simulink model "Model (1)"  (R2020a)
settings: Solver=VariableStepAuto  StartTime=0.0  StopTime=10.0  RelTol=1e-3
libraries: dspsigops x3, dsparch4 x3, dspswit3 x1, simulink_extras x1
settings Model: Creator=User  LastModifiedBy=Madhura

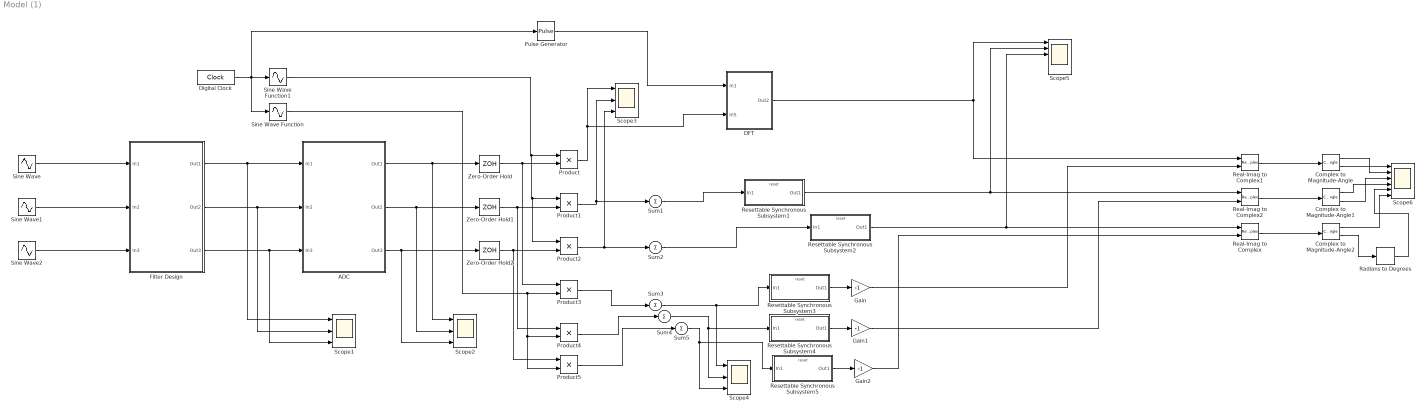
== system Model (1) ==
  ADC : Subsystem
  Complex to Magnitude-Angle : ComplexToMagnitudeAngle
  Complex to Magnitude-Angle1 : ComplexToMagnitudeAngle
  Complex to Magnitude-Angle2 : ComplexToMagnitudeAngle
  DFT : Subsystem
  Digital Clock : DigitalClock  SampleTime=0.001
  Filter Design : Subsystem
  Gain : Gain  Gain=-1
  Gain1 : Gain  Gain=-1
  Gain2 : Gain  Gain=-1
  Product{,1..5} (6 alike) : Product
  Pulse Generator : DiscretePulseGenerator  PulseType=Time based  TimeSource=Use external signal  Period=0.04  PulseWidth=50
  Radians to Degrees : simulink_extras/Transformations/Radians to Degrees
  Real-Imag to Complex : RealImagToComplex
  Real-Imag to Complex1 : RealImagToComplex
  Real-Imag to Complex2 : RealImagToComplex
  Resettable Synchronous Subsystem1 : Subsystem  TreatAsAtomicUnit=on
  Resettable Synchronous Subsystem2 : Subsystem  TreatAsAtomicUnit=on
  Resettable Synchronous Subsystem3 : Subsystem  TreatAsAtomicUnit=on
  Resettable Synchronous Subsystem4 : Subsystem  TreatAsAtomicUnit=on
  Resettable Synchronous Subsystem5 : Subsystem  TreatAsAtomicUnit=on
  Scope{1..4} (4 alike) : Scope  NumInputPorts=3
  Scope5 : Scope  NumInputPorts=6
  Scope6 : Scope  NumInputPorts=6
  Sine Wave : Sin  Amplitude=1.5  Frequency=2*pi*(53)  SampleTime=0
  Sine Wave Function : Sin  TimeSource=Use external signal  Frequency=2*pi/20  SampleTime=0
  Sine Wave Function1 : Sin  TimeSource=Use external signal  Frequency=2*pi/20  Phase=pi/2  SampleTime=0
  Sine Wave1 : Sin  Frequency=2*pi*50  SampleTime=0
  Sine Wave2 : Sin  Frequency=2*pi*50  Phase=-2*pi/3  SampleTime=0
  Sum1 : Sum  Inputs=+  CollapseMode=Specified dimension
  Sum{2..5} (4 alike) : Sum  Inputs=+
  Zero-Order Hold : ZeroOrderHold  SampleTime=-1
  Zero-Order Hold1 : ZeroOrderHold  SampleTime=-1
  Zero-Order Hold2 : ZeroOrderHold  SampleTime=-1
  wires:
  Sine Wave/1 -> Filter Design/1(In1)
  ADC/2(Out2) -> Zero-Order Hold1/1, Scope2/2
  Sine Wave1/1 -> Filter Design/2(In2)
  Filter Design/1(Out1) -> Scope1/1, ADC/1(In1)
  ADC/3(Out3) -> Zero-Order Hold2/1, Scope2/3
  ADC/1(Out1) -> Zero-Order Hold/1, Scope2/1
  Sine Wave2/1 -> Filter Design/3(In3)
  Filter Design/2(Out2) -> Scope1/2, ADC/2(In2)
  Filter Design/3(Out3) -> Scope1/3, ADC/3(In3)
  Zero-Order Hold/1 -> Product3/1, Product/2
  Zero-Order Hold1/1 -> Product4/1, Product1/2
  Zero-Order Hold2/1 -> Product5/1, Product2/2
  Digital Clock/1 -> Pulse Generator/1, Sine Wave Function1/1, Sine Wave Function/1
  Sine Wave Function1/1 -> Product2/1, Product1/1, Product/1
  Product1/1 -> Sum1/1, Scope3/2
  Product2/1 -> Sum2/1, Scope3/3
  Sine Wave Function/1 -> Product5/2, Product4/2, Product3/2
  Product3/1 -> Sum3/1
  Product4/1 -> Sum4/1
  Product5/1 -> Sum5/1
  Product/1 -> DFT/2(In5), Scope3/1
  Sum3/1 -> Resettable Synchronous Subsystem3/1(In1), Scope4/1
  Sum4/1 -> Resettable Synchronous Subsystem4/1(In1), Scope4/2
  Sum5/1 -> Resettable Synchronous Subsystem5/1(In1), Scope4/3
  Gain/1 -> Real-Imag to Complex1/2
  Gain1/1 -> Real-Imag to Complex2/2
  Gain2/1 -> Real-Imag to Complex/2
  Real-Imag to Complex1/1 -> Complex to Magnitude-Angle/1
  Real-Imag to Complex2/1 -> Complex to Magnitude-Angle1/1
  Real-Imag to Complex/1 -> Complex to Magnitude-Angle2/1
  Complex to Magnitude-Angle/2 -> Scope6/1
  Complex to Magnitude-Angle1/2 -> Scope6/3
  Complex to Magnitude-Angle/1 -> Scope6/2
  Complex to Magnitude-Angle1/1 -> Scope6/4
  Complex to Magnitude-Angle2/1 -> Scope6/6
  Resettable Synchronous Subsystem3/1(Out1) -> Gain/1
  Resettable Synchronous Subsystem1/1(Out1) -> Scope5/2, Real-Imag to Complex2/1
  Sum1/1 -> Resettable Synchronous Subsystem1/1(In1)
  Sum2/1 -> Resettable Synchronous Subsystem2/1(In1)
  Resettable Synchronous Subsystem2/1(Out1) -> Scope5/3, Real-Imag to Complex/1
  Resettable Synchronous Subsystem4/1(Out1) -> Gain1/1
  Resettable Synchronous Subsystem5/1(Out1) -> Gain2/1
  Complex to Magnitude-Angle2/2 -> Radians to Degrees/1
  Radians to Degrees/1 -> Scope6/5
  DFT/1(Out2) -> Scope5/1, Real-Imag to Complex1/1
  Pulse Generator/1 -> DFT/1(In1)

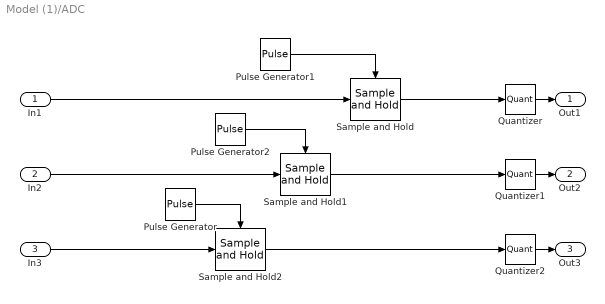
== system Model (1)/ADC ==
  In1 : Inport
  In2 : Inport  Port=2
  In3 : Inport  Port=3
  Pulse Generator : DiscretePulseGenerator  PulseType=Time based  Period=0.001  PulseWidth=5
  Pulse Generator1 : DiscretePulseGenerator  PulseType=Time based  Period=0.001  PulseWidth=5
  Pulse Generator2 : DiscretePulseGenerator  PulseType=Time based  Period=0.001  PulseWidth=5
  Quantizer : Quantizer  QuantizationInterval=0.1
  Quantizer1 : Quantizer  QuantizationInterval=0.1
  Quantizer2 : Quantizer  QuantizationInterval=0.1
  Sample and Hold : dspsigops/Sample and Hold  trig=Rising edge  initCond=0  latchinput=off
  Sample and Hold1 : dspsigops/Sample and Hold  trig=Rising edge  initCond=0  latchinput=off
  Sample and Hold2 : dspsigops/Sample and Hold  trig=Rising edge  initCond=0  latchinput=off
  Out1 : Outport
  Out2 : Outport  Port=2
  Out3 : Outport  Port=3
  wires:
  In1/1 -> Sample and Hold/1
  Sample and Hold2/1 -> Quantizer2/1
  Sample and Hold1/1 -> Quantizer1/1
  Pulse Generator1/1 -> Sample and Hold/Trigger
  In2/1 -> Sample and Hold1/1
  Pulse Generator/1 -> Sample and Hold2/Trigger
  Quantizer2/1 -> Out3/1
  Sample and Hold/1 -> Quantizer/1
  Pulse Generator2/1 -> Sample and Hold1/Trigger
  Quantizer/1 -> Out1/1
  Quantizer1/1 -> Out2/1
  In3/1 -> Sample and Hold2/1

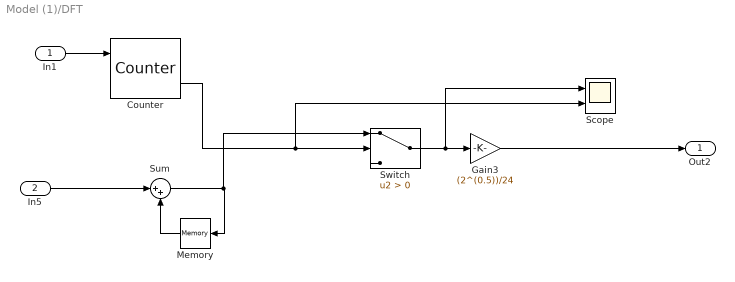
== system Model (1)/DFT ==
  In1 : Inport
  In5 : Inport  Port=2
  Counter : dspswit3/Counter  Direction=Up  CountEvent=Rising edge  CounterSize=User defined  MaxCount=20  InitialCount=0  Output=Count and Hit  HitValue=20  ResetInput=on  SamplesPerFrame=1  Ts=1  CntDtype=double  HitDtype=Logical
  Gain3 : Gain  Gain=(2^(0.5))/24
  Memory : Memory
  Scope : Scope  NumInputPorts=2
  Sum : Sum  Inputs=|++
  Switch : Switch  Criteria=u2 > Threshold
  Out2 : Outport
  wires:
  Gain3/1 -> Out2/1
  Switch/1 -> Scope/1, Gain3/1
  Sum/1 -> Switch/1, Memory/1
  In1/1 -> Counter/1
  Memory/1 -> Sum/2
  In5/1 -> Sum/1
  Counter/2 -> Scope/2, Switch/2

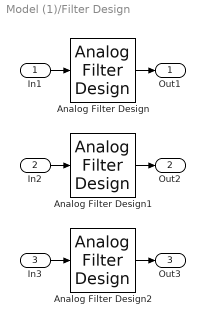
== system Model (1)/Filter Design ==
  In1 : Inport
  In2 : Inport  Port=2
  In3 : Inport  Port=3
  Analog Filter Design : dsparch4/Analog Filter Design  method=Butterworth  filttype=Lowpass  N=8  Wlo=2*pi*60  Whi=80  Rp=2  Rs=40
  Analog Filter Design1 : dsparch4/Analog Filter Design  method=Butterworth  filttype=Lowpass  N=8  Wlo=2*pi*60  Whi=80  Rp=2  Rs=40
  Analog Filter Design2 : dsparch4/Analog Filter Design  method=Butterworth  filttype=Lowpass  N=8  Wlo=2*pi*60  Whi=80  Rp=2  Rs=40
  Out1 : Outport
  Out2 : Outport  Port=2
  Out3 : Outport  Port=3
  wires:
  In2/1 -> Analog Filter Design1/1
  Analog Filter Design1/1 -> Out2/1
  In1/1 -> Analog Filter Design/1
  Analog Filter Design2/1 -> Out3/1
  In3/1 -> Analog Filter Design2/1
  Analog Filter Design/1 -> Out1/1

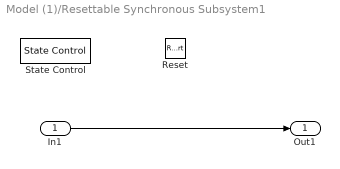
== system Model (1)/Resettable Synchronous Subsystem1 ==
  In1 : Inport
  Reset : ResetPort  DisableCoverage=on  ResetTriggerType=level hold
  State Control : StateControl  StateControl=Synchronous
  Out1 : Outport  VectorParamsAs1DForOutWhenUnconnected=off
  wires:
  In1/1 -> Out1/1

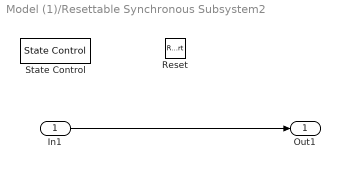
== system Model (1)/Resettable Synchronous Subsystem2 ==
  In1 : Inport
  Reset : ResetPort  DisableCoverage=on  ResetTriggerType=level hold
  State Control : StateControl  StateControl=Synchronous
  Out1 : Outport  VectorParamsAs1DForOutWhenUnconnected=off
  wires:
  In1/1 -> Out1/1

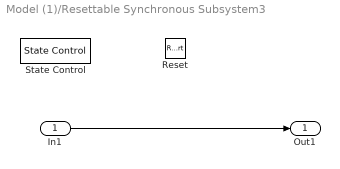
== system Model (1)/Resettable Synchronous Subsystem3 ==
  In1 : Inport
  Reset : ResetPort  DisableCoverage=on  ResetTriggerType=level hold
  State Control : StateControl  StateControl=Synchronous
  Out1 : Outport  VectorParamsAs1DForOutWhenUnconnected=off
  wires:
  In1/1 -> Out1/1

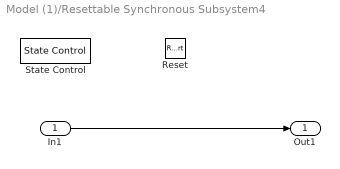
== system Model (1)/Resettable Synchronous Subsystem4 ==
  In1 : Inport
  Reset : ResetPort  DisableCoverage=on  ResetTriggerType=level hold
  State Control : StateControl  StateControl=Synchronous
  Out1 : Outport  VectorParamsAs1DForOutWhenUnconnected=off
  wires:
  In1/1 -> Out1/1

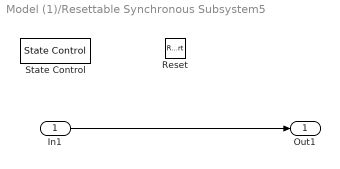
== system Model (1)/Resettable Synchronous Subsystem5 ==
  In1 : Inport
  Reset : ResetPort  DisableCoverage=on  ResetTriggerType=level hold
  State Control : StateControl  StateControl=Synchronous
  Out1 : Outport  VectorParamsAs1DForOutWhenUnconnected=off
  wires:
  In1/1 -> Out1/1
